simulink model "CoffeeVendingMachine"  (R2020a)
settings: Solver=VariableStepAuto  StartTime=0.0  StopTime=10.0  RelTol=1e-3
settings Model: Creator=Admin  LastModifiedBy=Admin

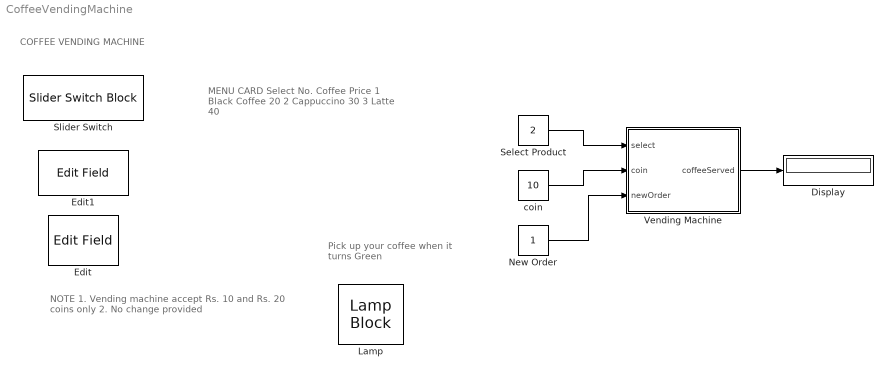
== system CoffeeVendingMachine ==
  note: Pick up your coffee
      | when it turns Green
  note: NOTE
      |
      | 1. Vending machine accept Rs. 10 and Rs. 20 coins only
      | 2. No change provided
  note: MENU CARD
      |
      | Select No. Coffee Price
      |
      | 1 Black Coffee 20
      | 2 Cappuccino 30
      | 3 Latte 40
  note: COFFEE VENDING MACHINE
  Display : Display
  Edit : EditField  ShowInitialText=on  Alignment=Center
  Edit1 : EditField  ShowInitialText=on  Alignment=Center
  Lamp : LampBlock
  New Order : Constant
  Select Product : Constant  Value=2
  Slider Switch : SliderSwitchBlock
      settings: Values={{'Off', 'On'}, [0 1]}
  Vending Machine : Stateflow chart  TreatAsAtomicUnit=on
  coin : Constant  Value=10
  wires:
  Select Product/1 -> Vending Machine/1(select)
  coin/1 -> Vending Machine/2(coin)
  Vending Machine/1(coffeeServed) -> Display/1
  New Order/1 -> Vending Machine/3(newOrder)

== stateflow chart CoffeeVendingMachine/Vending Machine ==
  settings: stateMachineType=MEALY_MACHINE
  state Start
  state SelectCoffee
  state WaitForMoney_1
  state Rupee10_1
  state Rupee20_1
  state Preparing
  state Served
  state Rupee10_2
  state Rupee30_2
  state WaitForMoney_2
  state Rupee20_2
  state Rupee40_3
  state Rupee10_3
  state Rupee30_3
  state WaitForMoney_3
  state Rupee20_3
  Served -> Start
  (default) -> Start
  Start -> SelectCoffee [order 1] : [newOrder == 1]
  Rupee10_1 -> Rupee20_1 : after(3,tick)[coin == 10]{coffeeServed = 0;}
  WaitForMoney_1 -> Rupee10_1 [order 1] : [coin == 10]{coffeeServed = 0;}
  SelectCoffee -> SelectCoffee [order 4] : [select == 0]
  Rupee20_1 -> Preparing : {coffeeServed = 0;}
  SelectCoffee -> WaitForMoney_1 [order 1] : [select == 1]
  Preparing -> Served : after(10,tick){coffeeServed=1;}
  SelectCoffee -> WaitForMoney_3 [order 3] : [select == 3]
  SelectCoffee -> WaitForMoney_2 [order 2] : [select == 2]
  Start -> Start [order 2] : [newOrder == 0]
  WaitForMoney_1 -> Rupee20_1 [order 2] : [coin == 20]{coffeeServed = 0;}
  Rupee30_2 -> Preparing : {coffeeServed == 0;}
  Rupee40_3 -> Preparing : {coffeeServed == 0;}
  WaitForMoney_1 -> WaitForMoney_1 [order 3] : [coin == 0]
  Rupee10_2 -> Rupee30_2 [order 2] : after(3,tick)[coin == 20]{coffeeServed = 0;}
  WaitForMoney_2 -> Rupee10_2 [order 1] : [coin == 10]{coffeeServed = 0;}
  Rupee10_2 -> Rupee20_2 [order 1] : after(3,tick)[coin == 10]{coffeeServed = 0;}
  Rupee20_2 -> Rupee30_2 : after(3,tick)[coin == 10]{coffeeServed = 0;}
  WaitForMoney_2 -> Rupee20_2 [order 2] : [coin == 20]{coffeeServed = 0;}
  WaitForMoney_2 -> WaitForMoney_2 [order 3] : [coin == 0]
  Rupee10_3 -> Rupee30_3 [order 2] : after(3,tick)[coin == 20]{coffeeServed = 0;}
  WaitForMoney_3 -> Rupee10_3 [order 1] : [coin == 10]{coffeeServed = 0;}
  Rupee10_3 -> Rupee20_3 [order 1] : after(3,tick)[coin == 10]{coffeeServed = 0;}
  Rupee30_3 -> Rupee40_3 : after(3,tick)[coin == 10]{coffeeServed = 0;}
  Rupee20_3 -> Rupee30_3 [order 1] : after(3,tick)[coin == 10]{coffeeServed = 0;}
  WaitForMoney_3 -> Rupee20_3 [order 2] : [coin == 20]{coffeeServed = 0;}
  WaitForMoney_3 -> WaitForMoney_3 [order 3] : [coin == 0]
  Rupee20_3 -> Rupee40_3 [order 2] : after(3,tick)[coin == 20]{coffeeServed = 0;}
  data: select input; coffeeServed output; coin input; newOrder input
